simulink model "pera_ros"  (R2022b)
settings: Solver=ode8  StartTime=0.0  StopTime=8  FixedStep=0.005  RelTol=1e-3
libraries: robotlib x7
settings Model: Creator=guillermo  LastModifiedBy=guillermo

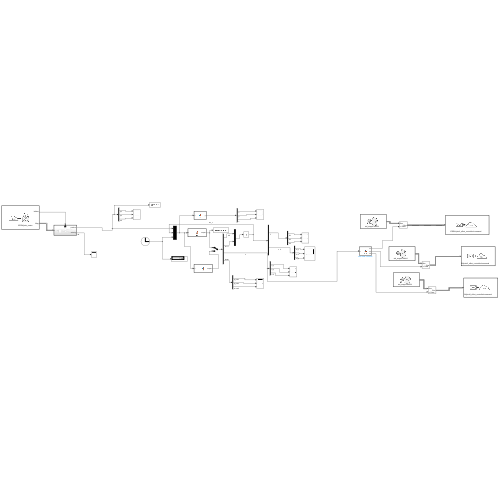
[thumbnail: Simulink's stored preview of the top-level diagram]
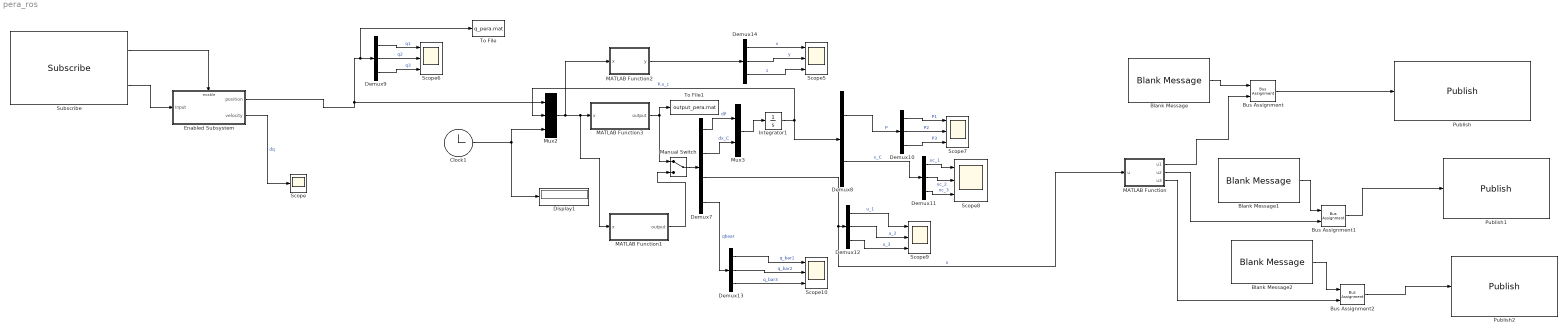
== system pera_ros ==
  Blank Message : robotlib/Blank Message  messageClass=Message  entityType=std_msgs/Float64  messageType=std_msgs/Float64  SampleTime=inf  legacyBusStruct=off
      settings: LibrarySourceBlock=roslib/ROS/Blank Message
  Blank Message1 : robotlib/Blank Message  messageClass=Message  entityType=std_msgs/Float64  messageType=std_msgs/Float64  SampleTime=inf  legacyBusStruct=off
      settings: LibrarySourceBlock=roslib/ROS/Blank Message
  Blank Message2 : robotlib/Blank Message  messageClass=Message  entityType=std_msgs/Float64  messageType=std_msgs/Float64  SampleTime=inf  legacyBusStruct=off
      settings: LibrarySourceBlock=roslib/ROS/Blank Message
  Bus Assignment : BusAssignment  AssignedSignals=Data
  Bus Assignment1 : BusAssignment  AssignedSignals=Data
  Bus Assignment2 : BusAssignment  AssignedSignals=Data
  Clock1 : Clock
  Demux{9..14} (6 alike) : Demux  Outputs=3
  Demux7 : Demux
  Demux8 : Demux  Outputs=2
  Display1 : Display
      settings: Decimation=30
  Enabled Subsystem : Subsystem  TreatAsAtomicUnit=on
  Integrator1 : Integrator  InitialCondition=[0;0;0;0;0;0]
  MATLAB Function : MATLAB Function  TreatAsAtomicUnit=on
  MATLAB Function1 : MATLAB Function  TreatAsAtomicUnit=on
  MATLAB Function2 : MATLAB Function  TreatAsAtomicUnit=on
  MATLAB Function3 : MATLAB Function  TreatAsAtomicUnit=on
  Manual Switch : ManualSwitch
  Mux2 : Mux  Inputs=3
  Mux3 : Mux  Inputs=2
  Publish : robotlib/Publish  topicSource=Select from ROS network  topic=/PERA/joint1_effort_controller/command  messageType=std_msgs/Float64  legacyBusStruct=off  messageQueueLength=1
      settings: LibrarySourceBlock=roslib/ROS/Publish
  Publish1 : robotlib/Publish  topicSource=Select from ROS network  topic=/PERA/joint2_effort_controller/command  messageType=std_msgs/Float64  legacyBusStruct=off  messageQueueLength=1
      settings: LibrarySourceBlock=roslib/ROS/Publish
  Publish2 : robotlib/Publish  topicSource=Select from ROS network  topic=/PERA/joint3_effort_controller/command  messageType=std_msgs/Float64  legacyBusStruct=off  messageQueueLength=1
      settings: LibrarySourceBlock=roslib/ROS/Publish
  Scope : Scope
  Scope{5..10} (6 alike) : Scope  NumInputPorts=3
  Subscribe : robotlib/Subscribe  topicSource=Select from ROS network  topic=/PERA/joint_states  messageType=sensor_msgs/JointState  SampleTime=-1  legacyBusStruct=off  messageQueueLength=1
      settings: LibrarySourceBlock=roslib/ROS/Subscribe
  To File : ToFile  Filename=q_pera.mat  MatrixName=q  SaveFormat=Timeseries
  To File1 : ToFile  Filename=output_pera.mat  MatrixName=q  SaveFormat=Timeseries
  wires:
  Blank Message1/1 -> Bus Assignment1/1
  Subscribe/2 -> Enabled Subsystem/1(Input)
  Bus Assignment/1 -> Publish/1
  Bus Assignment1/1 -> Publish1/1
  MATLAB Function/2(u2) -> Bus Assignment1/2
  Subscribe/1 -> Enabled Subsystem/Enable
  Blank Message/1 -> Bus Assignment/1
  Enabled Subsystem/1(position) -> To File/1, Demux9/1, Mux2/1
  MATLAB Function/1(u1) -> Bus Assignment/2
  Mux3/1 -> Integrator1/1
  Demux7/3 -> MATLAB Function/1(u), Demux12/1  "u"
  Demux13/2 -> Scope10/2  "q_bar2"
  MATLAB Function2/1(y) -> Demux14/1
  Demux11/2 -> Scope8/2  "xc_2"
  Demux7/4 -> Demux13/1  "qbaar"
  Demux9/1 -> Scope6/1  "q1"
  Demux12/2 -> Scope9/2  "u_2"
  Mux2/1 -> MATLAB Function2/1(x), MATLAB Function1/1(x), MATLAB Function3/1(x)
  Demux11/1 -> Scope8/1  "xc_1"
  Demux12/3 -> Scope9/3  "u_3"
  Demux10/1 -> Scope7/1  "P1"
  Integrator1/1 -> Mux2/2, Demux8/1  "P,x_c"
  Demux12/1 -> Scope9/1  "u_1"
  Demux14/1 -> Scope5/1  "x"
  Clock1/1 -> Mux2/3, Display1/1
  Demux13/3 -> Scope10/3  "q_bar3"
  Demux10/3 -> Scope7/3  "P3"
  Demux8/2 -> Demux11/1  "x_C"
  Demux11/3 -> Scope8/3  "xc_3"
  Demux10/2 -> Scope7/2  "P2"
  Demux14/2 -> Scope5/2  "y"
  Demux7/1 -> Mux3/1  "dP"
  Demux9/3 -> Scope6/3  "q3"
  MATLAB Function3/1(output) -> To File1/1, Manual Switch/1
  Demux14/3 -> Scope5/3  "z"
  Demux9/2 -> Scope6/2  "q2"
  Demux7/2 -> Mux3/2  "dx_C"
  Demux13/1 -> Scope10/1  "q_bar1"
  Demux8/1 -> Demux10/1  "P"
  Bus Assignment2/1 -> Publish2/1
  Blank Message2/1 -> Bus Assignment2/1
  MATLAB Function/3(u3) -> Bus Assignment2/2
  Enabled Subsystem/2(velocity) -> Scope/1  "dq"
  Manual Switch/1 -> Demux7/1
  MATLAB Function1/1(output) -> Manual Switch/2

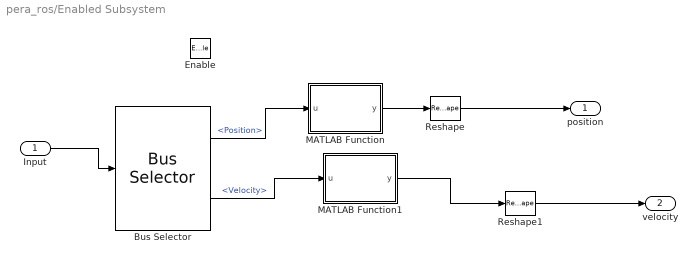
== system pera_ros/Enabled Subsystem ==
  Input : Inport
  Enable : EnablePort
  Bus Selector : BusSelector  OutputSignals=Position,Velocity
  MATLAB Function : MATLAB Function  TreatAsAtomicUnit=on
  MATLAB Function1 : MATLAB Function  TreatAsAtomicUnit=on
  Reshape : Reshape  OutputDimensionality=Column vector (2-D)
  Reshape1 : Reshape  OutputDimensionality=Column vector (2-D)
  position : Outport
  velocity : Outport  Port=2
  wires:
  Input/1 -> Bus Selector/1
  Bus Selector/1 -> MATLAB Function/1(u)  "<Position>"
  Bus Selector/2 -> MATLAB Function1/1(u)  "<Velocity>"
  MATLAB Function/1(y) -> Reshape/1
  MATLAB Function1/1(y) -> Reshape1/1
  Reshape/1 -> position/1
  Reshape1/1 -> velocity/1

== matlab function pera_ros/MATLAB Function1 ==
  data: x input; output output
function output = fcn(x)
q1 = x(1);
q2 = x(2);
q3 = x(3);
q = [q1; q2; q3]; % Joint positions
P1 = x(4);
P2 = x(5);
P3 = x(6);
P = [P1; P2; P3]; % Transformed momenta
x_c1 = x(7);
x_c2 = x(8);
x_c3 = x(9);
x_c = [x_c1; x_c2; x_c3]; % Artificial state
t = x(10);

 % Trajectory: Circle parameters
r = .2; % Radius of circle in meters
T = 30; % Period for drawing a circle in seconds
% Trajectory: Desired positions
q_d1 = 0;
q_d2 = asin(r/.48)*sin((2*pi/T)*t);
q_d3 = pi/2 - asin(r/.48)*cos((2*pi/T)*t);
q_d = [q_d1; q_d2; q_d3];

% Trajectory: Derivative of desired positions
dq_d1 = 0;
dq_d2 = (2*pi*asin((25*r)/12)*cos((2*pi*t)/T))/T;
dq_d3 = (2*pi*asin((25*r)/12)*sin((2*pi*t)/T))/T;
dq_d = [dq_d1; dq_d2; dq_d3];

% Error positions
q_bar = q - q_d;
 % Desired transformed momenta
P_d = [0; (2580715296368087*7616037329846245771365^(1/2)*pi*cos((2*pi*t)/15))...
    /6044629098073145873530880000;...
    (2580715296368087*195^(1/2)*pi*sin((2*pi*t)/15))/...
    4503599627370496000];
% Derivative of desired transformed momenta
dP_d = [0; ...
 -(2580715296368087*7616037329846245771365^(1/2)*pi^2*sin((2*pi*t)/15))/...
 45334718235548594051481600000;...
 (2580715296368087*195^(1/2)*pi^2*cos((2*pi*t)/15))/33776997205278720000];
% Error transformed momenta
P_bar = P - P_d;
% System matrices and gains
% Cholesky transform of the inertia matrix (Lower triangular, such that ..M^−1=T*T^T and P=T^T * p):
psi = [(26843545600*5^(1/2))/(1509102191936324763648*sin(q1)^2 + ...
110317174072316078125)^(1/2), 0, 0; 0, ...
(26843545600*7616037329846245771365^(1/2))/1523207465969249154273, 0; ...
-(26843545600*5^(1/2)*cos(q1))/(1619419366008640841773 - ...
1509102191936324763648*cos(q1)^2)^(1/2), 0, (20*195^(1/2))/39];
% Gyroscopic forces matrix
J2 = zeros(3,3);
alpha = [11;2;6]; % Chosen s.t. saturation limits cannot be exceeded
beta = [400; 100; 100];
K_c = diag([10 20 10]);
R_c = diag([1 1 1]);

 % Potential energies
dVdq = [6.17*sin(q1) + 1.57*cos(q3)*sin(q1) + 1.57*sin(q3)*cos(q1)*cos(q2); ...
-1.57*sin(q3)*sin(q1)*sin(q2); 1.57*sin(q3)*cos(q1) + ...
1.57*cos(q3)*cos(q2)*sin(q1)];

dV_ddq_d = [6.17*sin(q_d1) + 1.57*cos(q_d3)*sin(q_d1) + ...
1.57*sin(q_d3)*cos(q_d1)*cos(q_d2); -1.57*sin(q_d3)*sin(q_d1)*sin(q_d2); ...
1.57*sin(q_d3)*cos(q_d1) + 1.57*cos(q_d3)*cos(q_d2)*sin(q_d1)];

% Gradients of Hamiltonian
% H = 1/2*P_bar.'*P_bar + V(q)
dHdq = dVdq;
dHdP = P;

% Input
 z = q_bar + x_c;
dphidz = [alpha(1)*tanh(beta(1)*z(1)); alpha(2)*tanh(beta(2)*z(2)); ...
alpha(3)*tanh(beta(3)*z(3))];
u_bar = dVdq - dV_ddq_d - dphidz;
u_d = dV_ddq_d + (psi.')\dP_d;
u = u_bar + u_d;

% Time−derivatives of states
dq = psi*dHdP;
dP = (-psi.')*dHdq + J2*dHdP + (psi.')*u;
dx_c = -R_c*(K_c*x_c + dphidz);

% Output
output = [dP; dx_c; u; q_bar];

== matlab function pera_ros/MATLAB Function ==
  data: u input; u1 output; u2 output; u3 output
function [u1,u2,u3]= fcn(u)
u1=u(1)
u2=u(2)
u3=u(3)

== matlab function pera_ros/MATLAB Function3 ==
  data: x input; output output
function output = fcn(x)
q1 = x(1);
q2 = x(2)-pi/2;
q3 = x(3);
q = [q1; q2; q3]; % Joint positions
P1 = x(4);
P2 = x(5);
P3 = x(6);
P = [P1; P2; P3]; % Transformed momenta
x_c1 = x(7);
x_c2 = x(8);
x_c3 = x(9);
x_c = [x_c1; x_c2; x_c3]; % Artificial state
t = x(10);
f=2;

meat_traj_1=[-0.000036284073948  -0.000077250765261   0.009269322838493     0.063503649041252   0.202213438405126;
   0.002540649538898   0.017017342751491  -0.311916259369786    1.089737031376497  -0.742810373066684;
   0.000012714630135  -0.000831605507563   0.014637171764278    0.046334679434705  -0.003806852039210];

meat_traj_2= [   0.000018648205655  -0.000266683615187  -0.000064942947155   0.005523891626725   0.557579779700295;
  -0.002657243203306   0.042033190126571  -0.346074075959999    0.993697772726691  -0.330172442151600;
   0.000004012379566  -0.000026840071228  -0.000543042791407     0.003579291689338   0.111116145679972]
meat_traj_3 =[    0.000002363407310  -0.000062332770507  -0.007985074348800   0.049438330002750   1.748157173378859;
  -0.005896801988897   0.029605246290894   0.076992944079132  -0.479454695677252   2.323334189707329;
   0.000008974816343  -0.000050593018781  -0.009172508658181   0.055361636141147   1.949021584378424]

meat_trajectory_fit_q1_1=meat_traj_1(1,:);meat_trajectory_fit_q1_2=meat_traj_1(2,:);meat_trajectory_fit_q1_3=meat_traj_1(3,:);
meat_trajectory_fit_q2_1=meat_traj_2(1,:);meat_trajectory_fit_q2_2=meat_traj_2(2,:);meat_trajectory_fit_q2_3=meat_traj_2(3,:);
meat_trajectory_fit_q3_1=meat_traj_3(1,:);meat_trajectory_fit_q3_2=meat_traj_3(2,:);meat_trajectory_fit_q3_3=meat_traj_3(3,:);


%%
 % Trajectory: Circle parameters
r = .2; % Radius of circle in meters
T = 30; % Period for drawing a circle in seconds
% Trajectory: Desired positions
if t<f
    q_d1=0.2022;
    q_d2=0.5576;
    q_d3=1.7482;
    q_d = [q_d1; q_d2; q_d3];
elseif t >= f && t < f+2 
    t=t-f;
    q_d1 =polyval(meat_trajectory_fit_q1_1,t);
    q_d2 =polyval(meat_trajectory_fit_q2_1,t);
    q_d3 = polyval(meat_trajectory_fit_q3_1,t);
    q_d = [q_d1; q_d2; q_d3];
elseif t >= f+2 && t < f+4
    t=t-f;
     q_d1=polyval(meat_trajectory_fit_q1_2,t)
    q_d2 =polyval(meat_trajectory_fit_q2_2,t)
    q_d3 = polyval(meat_trajectory_fit_q3_2,t)
    q_d = [q_d1; q_d2; q_d3];
else
    t=t-f;
    q_d1=polyval(meat_trajectory_fit_q1_3,t)
    q_d2 =polyval(meat_trajectory_fit_q2_3,t)
    q_d3 = polyval(meat_trajectory_fit_q3_3,t)
    q_d = [q_d1; q_d2; q_d3];  
end

% Trajectory: Derivative of desired positions

if t<f
    dq_d1=0
    dq_d2=0
    dq_d3=0
    dq_d = [dq_d1; dq_d2; dq_d3];
    
elseif t >= f && t < f+2
    t=t-f;
    dq_d1=polyval(polyder(meat_trajectory_fit_q1_1),t)
    dq_d2=polyval(polyder(meat_trajectory_fit_q2_1),t)
    dq_d3=polyval(polyder(meat_trajectory_fit_q3_1),t)
    dq_d = [dq_d1; dq_d2; dq_d3];
elseif t >= f+2 && t < f+4
    t=t-f;
    dq_d1=polyval(polyder(meat_trajectory_fit_q1_2),t)
    dq_d2=polyval(polyder(meat_trajectory_fit_q2_2),t)
    dq_d3=polyval(polyder(meat_trajectory_fit_q3_2),t)
    dq_d = [dq_d1; dq_d2; dq_d3];
else
    t=t-f
    dq_d1=polyval(polyder(meat_trajectory_fit_q1_3),t)
    dq_d2=polyval(polyder(meat_trajectory_fit_q2_3),t)
    dq_d3=polyval(polyder(meat_trajectory_fit_q3_3),t)
    dq_d = [dq_d1; dq_d2; dq_d3]; 
end


% Error positions
q_bar = q - q_d;
 % Desired transformed momenta
P_d = [0; (2580715296368087*7616037329846245771365^(1/2)*pi*cos((2*pi*t)/15))...
    /6044629098073145873530880000;...
    (2580715296368087*195^(1/2)*pi*sin((2*pi*t)/15))/...
    4503599627370496000];
% Derivative of desired transformed momenta
dP_d = [0; ...
 -(2580715296368087*7616037329846245771365^(1/2)*pi^2*sin((2*pi*t)/15))/...
 45334718235548594051481600000;...
 (2580715296368087*195^(1/2)*pi^2*cos((2*pi*t)/15))/33776997205278720000];
% Error transformed momenta
P_bar = P - P_d;
% System matrices and gains
% Cholesky transform of the inertia matrix (Lower triangular, such that ..M^−1=T*T^T and P=T^T * p):
psi = [(26843545600*5^(1/2))/(1509102191936324763648*sin(q1)^2 + ...
110317174072316078125)^(1/2), 0, 0; 0, ...
(26843545600*7616037329846245771365^(1/2))/1523207465969249154273, 0; ...
-(26843545600*5^(1/2)*cos(q1))/(1619419366008640841773 - ...
1509102191936324763648*cos(q1)^2)^(1/2), 0, (20*195^(1/2))/39];

%%
psi_inv = inv(psi);

% Calculate the Lie bracket [Psi_i(q), Psi_j(q)]
Lie_bracket = zeros(3,3);
Lie_bracket(1,2) = psi(1,1)*psi(2,2) - psi(1,2)*psi(2,1);
Lie_bracket(1,3) = psi(1,1)*psi(3,2) - psi(1,2)*psi(3,1);
Lie_bracket(2,3) = psi(2,1)*psi(3,2) - psi(2,2)*psi(3,1);
Lie_bracket = Lie_bracket - Lie_bracket';

% Calculate the Jij matrix
J2 = -P'*psi_inv*Lie_bracket*psi_inv';
%%
% Gyroscopic forces matrix
J2 = zeros(3,3);
alpha = [12;3.5;6];
% Chosen s.t. saturation limits cannot be exceeded
beta = [400; 200; 220];
K_c = diag([100 100 200]);
R_c = 10^(0)*diag([1 0.1 4.5500]);

alpha = [12;3.5;6]; % Chosen s.t. saturation limits cannot be exceeded
beta = [400; 100; 120];
K_c = diag([30 20 200]);
R_c = 10^(-4)*diag([1 0.1 4500])

 % Potential energies
dVdq = [6.17*sin(q1) + 1.57*cos(q3)*sin(q1) + 1.57*sin(q3)*cos(q1)*cos(q2); ...
-1.57*sin(q3)*sin(q1)*sin(q2); 1.57*sin(q3)*cos(q1) + ...
1.57*cos(q3)*cos(q2)*sin(q1)];

dV_ddq_d = [6.17*sin(q_d1) + 1.57*cos(q_d3)*sin(q_d1) + ...
1.57*sin(q_d3)*cos(q_d1)*cos(q_d2); -1.57*sin(q_d3)*sin(q_d1)*sin(q_d2); ...
1.57*sin(q_d3)*cos(q_d1) + 1.57*cos(q_d3)*cos(q_d2)*sin(q_d1)];

% Gradients of Hamiltonian
% H = 1/2*P_bar.'*P_bar + V(q)
dHdq = dVdq;
dHdP = P;

% Input
 z = q_bar + x_c;
dphidz = [alpha(1)*tanh(beta(1)*z(1)); alpha(2)*tanh(beta(2)*z(2)); ...
alpha(3)*tanh(beta(3)*z(3))];
u_bar = dVdq - dV_ddq_d - dphidz;
u_d = dV_ddq_d + (psi.')\dP_d;
u = u_bar + u_d;

% Time−derivatives of states
dq = psi*dHdP;
dP = (-psi.')*dHdq + J2*dHdP + (psi.')*u;
dx_c = -R_c*(K_c*x_c + dphidz);

% Output
output = [dP; dx_c; u; q_bar];

== matlab function pera_ros/Enabled Subsystem/MATLAB Function ==
  data: u input; y output
function y = fcn(u)
y=[0;0;0]

y(1)=u(1)
y(2)=u(2)
y(3)=u(3)

== matlab function pera_ros/Enabled Subsystem/MATLAB Function1 ==
  data: u input; y output
function y = fcn(u)
y=[0;0;0]

y(1)=u(1)
y(2)=u(2)
y(3)=u(3)

== matlab function pera_ros/MATLAB Function2 ==
  data: x input; y output
function y = fcn(x)
q1 = x(1);
q2 = x(2);
q3 = x(3);
q = [q1; q2; q3]; % Joint positions
P1 = x(4);
P2 = x(5);
P3 = x(6);
P = [P1; P2; P3]; % Transformed momenta
x_c1 = x(7);
x_c2 = x(8);
x_c3 = x(9);
x_c = [x_c1; x_c2; x_c3]; % Artificial state
t = x(10);
T_2=2;

trajectory_x_pera = [0.0000   -0.0060    0.1036   -0.3548    0.5929];
trajectory_y_pera =[ -0.0000    0.0000    0.0000    0.0500   -0.1500];
   if t<2
       t=0
       x_meat_pera=0.44;
       y_meat_pera=0.25;
       z_meat_pera= -0.15+(0.1/T_2)*t;
       end_effector = [x_meat_pera;y_meat_pera;z_meat_pera];
   elseif t >= 2 && t < 4
       t=t-2
       x_meat_pera=0.44;
       y_meat_pera=0.25;
       z_meat_pera= -0.15+(0.1/T_2)*t;
       end_effector = [x_meat_pera;y_meat_pera;z_meat_pera];
   elseif t >= 4 && t < 6
       t=t-2
        x_meat_pera=0.44;
        %y_meat_pera(i)=new_pos((i-200),1)
        y_meat_pera=polyval(trajectory_x_pera,t);
        %z_meat_pera(i)= new_pos((i-200),2)
        z_meat_pera=polyval(trajectory_y_pera,t); 
        end_effector = [x_meat_pera;y_meat_pera;z_meat_pera]

   else
        t=t-2
        x_meat_pera=0.44;
        y_meat_pera= 0.45;
        z_meat_pera=-0.15+(0.1/T_2)*t;
        end_effector = [x_meat_pera;y_meat_pera;z_meat_pera]

    
    end


q_traj_1 = 0.32*sin(q1) + 0.48*cos(q3)*sin(q1) - 0.000000000000000029391523179536476972170336707002*sin(q1)*sin(q2)*sin(q3) + 0.48*cos(q1)*cos(q2)*sin(q3) + 0.000000000000000029391523179536476972170336707002*cos(q1)*cos(q3)*sin(q2) + 1.7997117391942292015966170542954e-33*cos(q2)*cos(q3)*sin(q1)
q_traj_2=7.2925960287368928606091375295513e-65*sin(q3)*(6.5820182292848241686198767302294e+63*sin(q2) + 24678615572537722894699718508544.0*cos(q1)*sin(q2) + 4.0303237782057736850134851968965e+47*cos(q2)*sin(q1)) - 0.000000000000000029391523179510182266047057330998*cos(q3)*(cos(q1) - 1.0) - 4.4654271920337339859627207990276e-81*cos(q3)*(6.5820182292848241686198767302294e+63*cos(q2) + 24678615572537722894699718508544.0*cos(q1)*cos(q2) - 4.0303237782057736850134851968965e+47*sin(q1)*sin(q2)) - 0.000000000000000019594348786373779575987468057696*cos(q1) + 0.000000000000000019594348786373779575987468057696;
q_traj_3=3.6227849345677337978887464278104e-49*cos(q3)*(4967757600021511.0*cos(q2) - 4967757600021511.0*cos(q1)*cos(q2) + 81129638414606681695789005144064.0*sin(q1)*sin(q2)) - 7.2925960287435254380594500630236e-65*cos(q3)*(6.5820182292848241686198767302294e+63*cos(q1) + 24678615572571482867467662723121.0) - 0.32*cos(q1) + 5.9164567891575885405879642396209e-33*sin(q3)*(4967757600021511.0*cos(q1)*sin(q2) - 4967757600021511.0*sin(q2) + 81129638414606681695789005144064.0*cos(q2)*sin(q1)) - 1.1998078261294861193028074754981e-33

q_traj = [q_traj_1;q_traj_2;q_traj_3];
error = q_traj-end_effector;

y = error;
